simulink model "Sim_localization"  (R2024b)
settings: Solver=VariableStepAuto  StartTime=0.0  StopTime=total_time  MaxStep=0.001  RelTol=1e-3
values from neighbouring files (symbols this model uses):
  d = 0.165    [init_localization.m]
  d_actual = 0.164    [init_localization.m]
  mode = 2    [init_localization.m]
  omega_trj = 2*pi    (= 6.28318530718)    [init_localization.m]
  PHI_INIT = [0;0]    [init_localization.m]
  Q_INIT = [q(1,1), q(2,1), q(3,1)]'    [init_localization.m]
  r = 0.03    [init_localization.m]
  R = 0.4    [init_localization.m]
  r_actual = 0.031    [init_localization.m]
  T_s = 0.001    [init_localization.m]
  total_time = 20    [init_localization.m]
  zoh_activation = 2    [init_localization.m]
undefined symbols (not defined in the file or in its folder): D, P_INIT_EKF, Q_INIT_LOC, R_2, R_4, Z_INIT_EKF
libraries: dspsigops x2
settings Model: Creator=alberto  LastModifiedBy=Riccardo
settings RTWCC: GPUComputeCapability=3.5

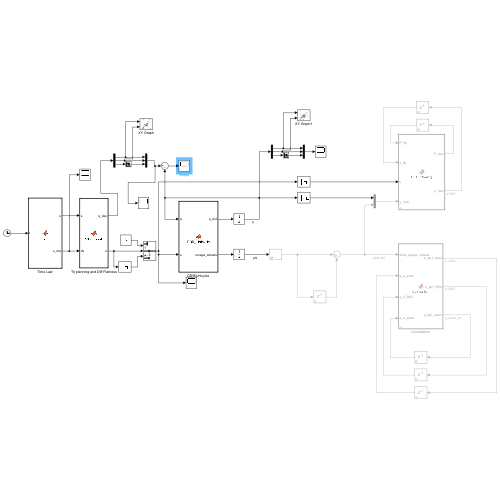
[thumbnail: Simulink's stored preview of the top-level diagram]
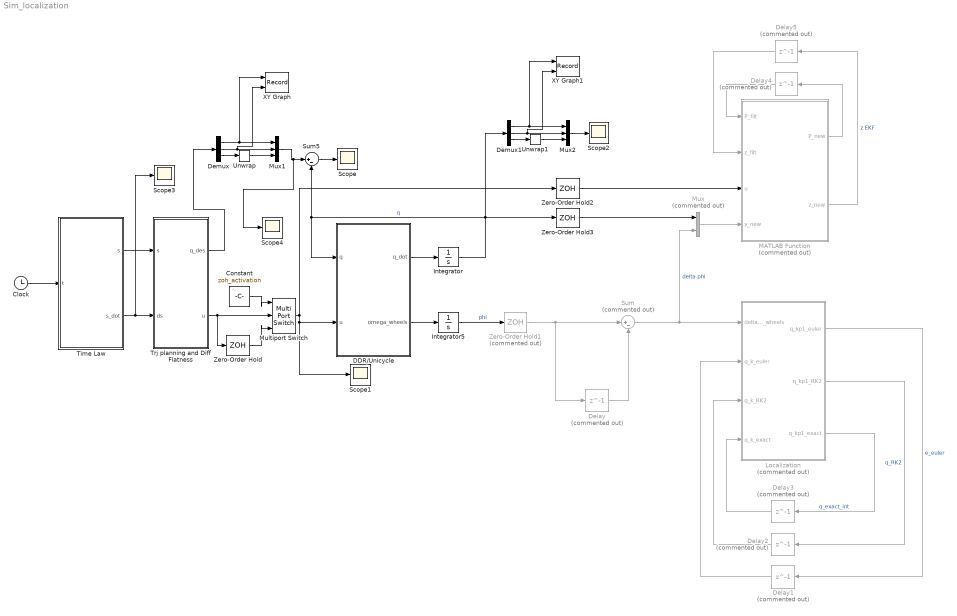
== system Sim_localization ==
  Clock : Clock
  Constant : Constant  Value=zoh_activation
  DDR/Unicycle : MATLAB Function  TreatAsAtomicUnit=on
  Delay : Delay  Commented=on  DelayLength=1  InitialCondition=[0;0]  SampleTime=T_s
  Delay1 : Delay  Commented=on  DelayLength=1  InitialCondition=Q_INIT_LOC
  Delay2 : Delay  Commented=on  DelayLength=1  InitialCondition=Q_INIT_LOC
  Delay3 : Delay  Commented=on  DelayLength=1  InitialCondition=Q_INIT_LOC
  Delay4 : Delay  Commented=on  DelayLength=1  InitialCondition=P_INIT_EKF  SampleTime=T_s
  Delay5 : Delay  Commented=on  DelayLength=1  InitialCondition=Z_INIT_EKF  SampleTime=T_s
  Demux : Demux  Outputs=3
  Demux1 : Demux  Outputs=3
  Integrator : Integrator  InitialCondition=Q_INIT
  Integrator5 : Integrator  InitialCondition=PHI_INIT
  Localization : MATLAB Function  Commented=on  TreatAsAtomicUnit=on
  MATLAB Function : MATLAB Function  Commented=on  TreatAsAtomicUnit=on
  Multiport Switch : MultiPortSwitch  Inputs=2  SaturateOnIntegerOverflow=off  InputSameDT=off
  Mux : Mux  Commented=on  Inputs=2
  Mux1 : Mux  Inputs=3
  Mux2 : Mux  Inputs=3
  Scope{,1..4} (5 alike) : Scope
  Sum : Sum  Commented=on  Inputs=|+-
  Sum5 : Sum  Inputs=|+-
  Time Law : MATLAB Function  TreatAsAtomicUnit=on
  Trj planning and Diff Flatness : MATLAB Function  TreatAsAtomicUnit=on
  Unwrap : dspsigops/Unwrap  tol=pi  InputProcessing=Columns as channels (frame based)  running=off
  Unwrap1 : dspsigops/Unwrap  tol=pi  InputProcessing=Columns as channels (frame based)  running=off
  XY Graph : Record  FileSettingsInternal="{\"entries\":[{\"content\":{\"excelSettings\":{\"content\":{},\"type\":\"Streamout.ExcelSettings\"}},\"type\":\"Streamout.FileSettingStorage\",\"uuid\":\"\"}],\"packageUris\":[\"http:\\/\\/schema.mathworks.com\\/mf0\\/streamout_blocks\\/R2020a\"],\"version\":\"1.0\"}"  Layout=[1 1]  SignalsInternal="{\"entries\":[{\"content\":{\"signals\":[{\"content\":{\"blockPath\":[],\"dimensions\":[1,1],\"domain\":\"\",\"lineColor\":\"#a2142f\",\"plots\":[ 1 ],\"port\":1,\"sid\":[\"\"],\"signalID\":1,\"signalName\":\"Demux:1\"},\"type\":\"RecordBlkView.Signal\",\"uuid\":\"\"},{\"content\":{\"blockPath\":[],\"dimensions\":[1,1],\"domain\":\"\",\"lineColor\":\"#139fff\",\"plots\":[ 1 ],\"port\":2,\"sid\":[\"\"],\"signalID\":2,\"signalName\":\"Demux:2\"},\"type\":\"RecordBlkView.Signal\",\"uuid\":\"\"}]},\"type\":\"RecordBlkView.InputSignals\",\"uuid\":\"\"}],\"packageUris\":[\"http:\\/\\/schema.mathworks.com\\/mf0\\/streamout_blocks\\/R2020a\"],\"version\":\"1.0\"}"  VisualizationBindings="{\"xyplotplugin\":{\"info\":[{\"series\":[{\"bindingParametersList\":[{\"parameter\":\"X-Axis\",\"signalID\":1,\"signalName\":\"Demux:1\"},{\"parameter\":\"Y-Axis\",\"signalID\":2,\"signalName\":\"Demux:2\"}],\"seriesID\":0}],\"subplotID\":1}]}}"  CompatibilityTag=XY
  XY Graph1 : Record  FileSettingsInternal="{\"entries\":[{\"content\":{\"excelSettings\":{\"content\":{},\"type\":\"Streamout.ExcelSettings\"}},\"type\":\"Streamout.FileSettingStorage\",\"uuid\":\"\"}],\"packageUris\":[\"http:\\/\\/schema.mathworks.com\\/mf0\\/streamout_blocks\\/R2020a\"],\"version\":\"1.0\"}"  Layout=[1 1]  SignalsInternal="{\"entries\":[{\"content\":{\"signals\":[{\"content\":{\"blockPath\":[],\"dimensions\":[1,1],\"domain\":\"\",\"lineColor\":\"#a2142f\",\"plots\":[ 1 ],\"port\":1,\"sid\":[\"\"],\"signalID\":1,\"signalName\":\"Demux1:1\"},\"type\":\"RecordBlkView.Signal\",\"uuid\":\"\"},{\"content\":{\"blockPath\":[],\"dimensions\":[1,1],\"domain\":\"\",\"lineColor\":\"#139fff\",\"plots\":[ 1 ],\"port\":2,\"sid\":[\"\"],\"signalID\":2,\"signalName\":\"Demux1:2\"},\"type\":\"RecordBlkView.Signal\",\"uuid\":\"\"}]},\"type\":\"RecordBlkView.InputSignals\",\"uuid\":\"\"}],\"packageUris\":[\"http:\\/\\/schema.mathworks.com\\/mf0\\/streamout_blocks\\/R2020a\"],\"version\":\"1.0\"}"  VisualizationBindings="{\"xyplotplugin\":{\"info\":[{\"series\":[{\"bindingParametersList\":[{\"parameter\":\"X-Axis\",\"signalID\":1,\"signalName\":\"Demux1:1\"},{\"parameter\":\"Y-Axis\",\"signalID\":2,\"signalName\":\"Demux1:2\"}],\"seriesID\":0}],\"subplotID\":1}]}}"  CompatibilityTag=XY
  Zero-Order Hold : ZeroOrderHold  SampleTime=T_s
  Zero-Order Hold1 : ZeroOrderHold  Commented=on  SampleTime=T_s
  Zero-Order Hold2 : ZeroOrderHold  SampleTime=T_s
  Zero-Order Hold3 : ZeroOrderHold  SampleTime=T_s
  wires:
  Clock/1 -> Time Law/1(t)
  Zero-Order Hold1/1 -> Sum/1, Delay/1
  Delay/1 -> Sum/2
  Delay1/1 -> Localization/2(q_k_euler)
  Sum/1 -> Mux/2, Localization/1(delta_angles_wheels)  "delta phi"
  Localization/1(q_kp1_euler) -> Delay1/1  "e_euler"
  Integrator/1 -> Demux1/1, Sum5/2, DDR/Unicycle/1(q), Zero-Order Hold3/1  "q"
  Delay3/1 -> Localization/4(q_k_exact)
  Delay2/1 -> Localization/3(q_k_RK2)
  Localization/2(q_kp1_RK2) -> Delay2/1  "q_RK2"
  Localization/3(q_kp1_exact) -> Delay3/1  "q_exact_int"
  Time Law/1(s) -> Trj planning and Diff Flatness/1(s)
  Time Law/2(s_dot) -> Scope3/1, Trj planning and Diff Flatness/2(ds)
  DDR/Unicycle/1(q_dot) -> Integrator/1
  Trj planning and Diff Flatness/1(q_des) -> Demux/1
  DDR/Unicycle/2(omega_wheels) -> Integrator5/1
  Integrator5/1 -> Zero-Order Hold1/1  "phi"
  MATLAB Function/1(P_new) -> Delay4/1
  Delay4/1 -> MATLAB Function/1(P_filt)
  Delay5/1 -> MATLAB Function/2(z_filt)
  MATLAB Function/2(z_new) -> Delay5/1  "z EKF"
  Mux/1 -> MATLAB Function/4(y_new)
  Trj planning and Diff Flatness/2(u) -> Zero-Order Hold/1, Multiport Switch/2
  Sum5/1 -> Scope/1
  Demux/3 -> Unwrap/1
  Multiport Switch/1 -> Scope1/1, DDR/Unicycle/2(u), Zero-Order Hold2/1
  Mux1/1 -> Scope4/1, Sum5/1
  Unwrap/1 -> Mux1/3
  Demux/2 -> XY Graph/2, Mux1/2
  Demux/1 -> XY Graph/1, Mux1/1
  Unwrap1/1 -> Mux2/3
  Demux1/3 -> Unwrap1/1
  Demux1/2 -> XY Graph1/2, Mux2/2
  Demux1/1 -> XY Graph1/1, Mux2/1
  Mux2/1 -> Scope2/1
  Zero-Order Hold3/1 -> Mux/1
  Zero-Order Hold2/1 -> MATLAB Function/3(u)
  Zero-Order Hold/1 -> Multiport Switch/3
  Constant/1 -> Multiport Switch/1

== matlab function Sim_localization/Time Law ==
  data: t input; s output; s_dot output; total_time parameter; mode parameter
function [s, s_dot] = fcn(t,total_time, mode)
s=0;
s_dot=0;
if mode==1%if mode =1 costasnt time law else trapezoidal
    s_dot = 1/total_time;
    s=t/total_time;
else
    Ta=0.5;% acceleration/dec time 10% of total
    Tc=9;%time of costant time

    Vc=1/(Ta+Tc);% velocità costante
    a=Vc/Ta;% acceleration
    
    switch 1 %formula on the slide
        case t<Ta
            s_dot=a*t;
            s=(a*(t^2))/2;

        case (t>=Ta)&&(t<(Tc+Ta))
            s_dot=Vc;
            s=(a*(Ta^2))/2+Vc*(t-Ta);

        case (t>=(Tc+Ta))&&(t<(Tc+2*Ta))
            s_dot=Vc-a*(t-Ta-Tc);
            s=(a*(Ta^2))/2+Vc*Tc+Vc*(t-Ta-Tc)-a*(t-Ta-Tc)^2/2;

        case t>=(Tc+2*Ta)
            s_dot=0;
            s=1;
    end

end

== matlab function Sim_localization/DDR//Unicycle ==
  data: q input; u input; q_dot output; omega_wheels output; d_actual parameter; r_actual parameter
function [q_dot, omega_wheels] = DDR_Unicycle(q, u, d_actual, r_actual)
v = u(1);
omega = u(2);

q_dot = [cos(q(3))*v; sin(q(3))*v; omega];

%evaluation of speed wheels
omega_L = (v - d_actual*omega) / (2*r_actual);
omega_R = (v + d_actual*omega) / (2*r_actual);
omega_wheels=[omega_R; omega_L];

== matlab function Sim_localization/Trj planning and Diff Flatness ==
  data: q_des output; s input; u output; ds input; R parameter; omega_trj parameter
function [q_des, u] = get_inputs(s, ds,R,omega_trj)

x=R*sin(2*omega_trj.*s);
y=R*sin(omega_trj.*s);

x_dot = R*2*omega_trj*cos(2*omega_trj.*s);
y_dot = R*omega_trj*cos(omega_trj.*s);

x_ddot = R*4*omega_trj*omega_trj*(-sin(2*omega_trj.*s));
y_ddot = R*omega_trj*omega_trj*(-sin(omega_trj.*s));

theta = atan2(y_dot,x_dot);

%   v
v = ds.*sqrt(y_dot.^2 + x_dot.^2);

%   omega
w = ds.*(x_dot.*y_ddot - y_dot.*x_ddot)./(y_dot.^2 + x_dot.^2);
    
q_des = [x; y; theta];
u = [v; w];

== matlab function Sim_localization/Localization ==
  data: delta_angles_wheels input; q_k_euler input; q_k_RK2 input; q_k_exact input; r parameter; d parameter; q_kp1_euler output; T_s parameter; q_kp1_RK2 output; q_kp1_exact output
function [q_kp1_euler, q_kp1_RK2, q_kp1_exact] = localization(delta_angles_wheels, q_k_euler, q_k_RK2, q_k_exact, r, d, T_s)

== matlab function Sim_localization/MATLAB Function ==
  data: P_filt input; P_new output; z_filt input; z_new output; u input; y_new input; D parameter; R_2 parameter; R_4 parameter; T_s parameter; r parameter; d parameter
function [P_new, z_new] = EKF_filtering(P_filt, z_filt, u, y_new, D, R_2, R_4, T_s, r, d)
